simulink model "Phase_Space_Test"  (R2022b)
settings: Solver=VariableStepAuto  StartTime=0.0  StopTime=sim_time  RelTol=1e-3
undefined symbols (not defined in the file or in its folder): icl, icn
settings Model: Creator=gotta  LastModifiedBy=gotta

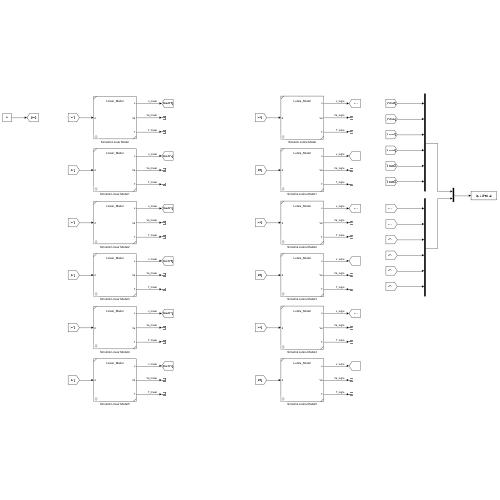
[thumbnail: Simulink's stored preview of the top-level diagram]
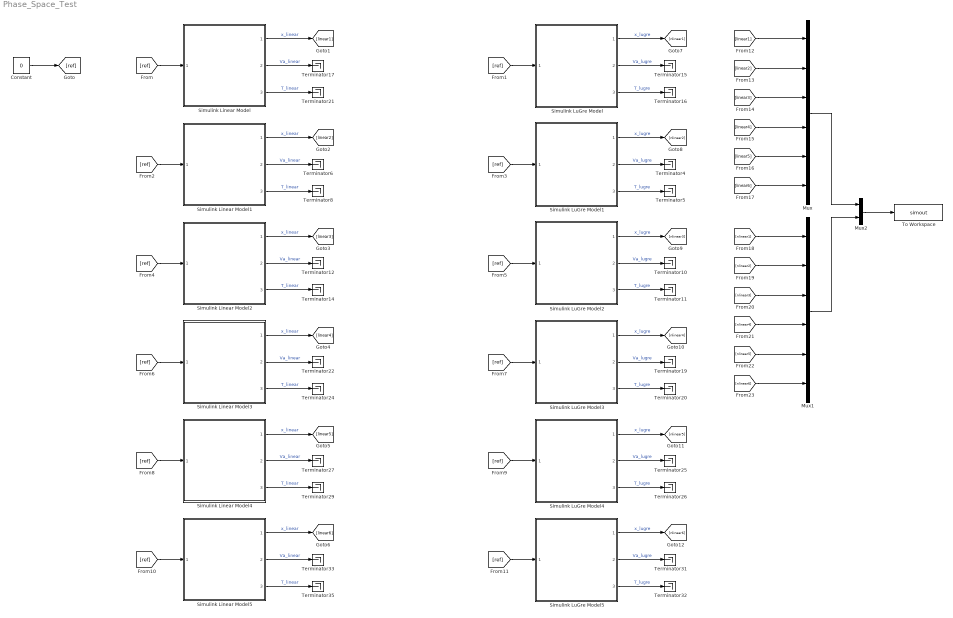
== system Phase_Space_Test ==
  Constant : Constant  Value=0
  Mux : Mux  Inputs=6
  Mux1 : Mux  Inputs=6
  Mux2 : Mux  Inputs=2
  Simulink Linear Model : Subsystem  ReferencedSubsystem=Linear_Model  motor_model=motor  initial_conditions=icl(:, 1)
  Simulink Linear Model1 : Subsystem  ReferencedSubsystem=Linear_Model  motor_model=motor  initial_conditions=icl(:, 2)
  Simulink Linear Model2 : Subsystem  ReferencedSubsystem=Linear_Model  motor_model=motor  initial_conditions=icl(:, 3)
  Simulink Linear Model3 : Subsystem  ReferencedSubsystem=Linear_Model  motor_model=motor  initial_conditions=icl(:, 4)
  Simulink Linear Model4 : Subsystem  ReferencedSubsystem=Linear_Model  motor_model=motor  initial_conditions=icl(:, 5)
  Simulink Linear Model5 : Subsystem  ReferencedSubsystem=Linear_Model  motor_model=motor  initial_conditions=icl(:, 6)
  Simulink LuGre Model : Subsystem  ReferencedSubsystem=LuGre_Model  motor_model=motor  initial_conditions=icn(:, 1)
  Simulink LuGre Model1 : Subsystem  ReferencedSubsystem=LuGre_Model  motor_model=motor  initial_conditions=icn(:, 2)
  Simulink LuGre Model2 : Subsystem  ReferencedSubsystem=LuGre_Model  motor_model=motor  initial_conditions=icn(:, 3)
  Simulink LuGre Model3 : Subsystem  ReferencedSubsystem=LuGre_Model  motor_model=motor  initial_conditions=icn(:, 4)
  Simulink LuGre Model4 : Subsystem  ReferencedSubsystem=LuGre_Model  motor_model=motor  initial_conditions=icn(:, 5)
  Simulink LuGre Model5 : Subsystem  ReferencedSubsystem=LuGre_Model  motor_model=motor  initial_conditions=icn(:, 6)
  Terminator{4..6,8,10..12,14..17,19..22,24..27,29,31..33,35} (24 alike) : Terminator
  To Workspace : ToWorkspace  VariableName=simout  SaveFormat=Structure With Time  SampleTime=1e-3
  wires:
  Simulink Linear Model/3 -> Terminator21/1  "T_linear"
  Simulink Linear Model/1 -> [linear1]  "x_linear"
  Simulink Linear Model/2 -> Terminator17/1  "Va_linear"
  Simulink LuGre Model/3 -> Terminator16/1  "T_lugre"
  Simulink LuGre Model/2 -> Terminator15/1  "Va_lugre"
  Simulink LuGre Model/1 -> [nlinear1]  "x_lugre"
  Constant/1 -> [ref]
  [ref] -> Simulink Linear Model/1
  [ref] -> Simulink LuGre Model/1
  [ref] -> Simulink LuGre Model1/1
  [ref] -> Simulink Linear Model1/1
  Simulink LuGre Model1/1 -> [nlinear2]  "x_lugre"
  Simulink LuGre Model1/2 -> Terminator4/1  "Va_lugre"
  Simulink LuGre Model1/3 -> Terminator5/1  "T_lugre"
  Simulink Linear Model1/2 -> Terminator6/1  "Va_linear"
  Simulink Linear Model1/1 -> [linear2]  "x_linear"
  Simulink Linear Model1/3 -> Terminator8/1  "T_linear"
  Simulink Linear Model3/3 -> Terminator24/1  "T_linear"
  Simulink Linear Model3/1 -> [linear4]  "x_linear"
  Simulink Linear Model3/2 -> Terminator22/1  "Va_linear"
  Simulink LuGre Model3/3 -> Terminator20/1  "T_lugre"
  Simulink LuGre Model3/2 -> Terminator19/1  "Va_lugre"
  Simulink LuGre Model3/1 -> [nlinear4]  "x_lugre"
  [ref] -> Simulink Linear Model3/1
  [ref] -> Simulink LuGre Model3/1
  [ref] -> Simulink LuGre Model2/1
  [ref] -> Simulink Linear Model2/1
  Simulink LuGre Model2/1 -> [nlinear3]  "x_lugre"
  Simulink LuGre Model2/2 -> Terminator10/1  "Va_lugre"
  Simulink LuGre Model2/3 -> Terminator11/1  "T_lugre"
  Simulink Linear Model2/2 -> Terminator12/1  "Va_linear"
  Simulink Linear Model2/1 -> [linear3]  "x_linear"
  Simulink Linear Model2/3 -> Terminator14/1  "T_linear"
  Simulink Linear Model4/3 -> Terminator29/1  "T_linear"
  Simulink Linear Model4/1 -> [linear5]  "x_linear"
  Simulink Linear Model4/2 -> Terminator27/1  "Va_linear"
  Simulink LuGre Model4/3 -> Terminator26/1  "T_lugre"
  Simulink LuGre Model4/2 -> Terminator25/1  "Va_lugre"
  Simulink LuGre Model4/1 -> [nlinear5]  "x_lugre"
  [ref] -> Simulink Linear Model4/1
  [ref] -> Simulink LuGre Model4/1
  [ref] -> Simulink LuGre Model5/1
  [ref] -> Simulink Linear Model5/1
  Simulink LuGre Model5/1 -> [nlinear6]  "x_lugre"
  Simulink LuGre Model5/2 -> Terminator31/1  "Va_lugre"
  Simulink LuGre Model5/3 -> Terminator32/1  "T_lugre"
  Simulink Linear Model5/2 -> Terminator33/1  "Va_linear"
  Simulink Linear Model5/1 -> [linear6]  "x_linear"
  Simulink Linear Model5/3 -> Terminator35/1  "T_linear"
  [linear1] -> Mux/1
  [linear2] -> Mux/2
  [linear3] -> Mux/3
  [linear4] -> Mux/4
  [linear5] -> Mux/5
  [linear6] -> Mux/6
  [nlinear6] -> Mux1/6
  [nlinear5] -> Mux1/5
  [nlinear4] -> Mux1/4
  [nlinear3] -> Mux1/3
  [nlinear2] -> Mux1/2
  [nlinear1] -> Mux1/1
  Mux/1 -> Mux2/1
  Mux1/1 -> Mux2/2
  Mux2/1 -> To Workspace/1
